simulink model "sim_track"  (Simulink 6.2)
settings: Solver=ode45  StartTime=0.0  StopTime=Tmax  MaxStep=0.01*T  RelTol=1e-6
undefined symbols (not defined in the file or in its folder): dF, dFo, dG, dK, dQ, dQu, dR, nF, nFo, nG, nK, nQ, nQu, nR, T, tauF, tauG, tauQ, tauQu, tauR
settings Model: LastModifiedBy=Administrator
settings DataIOCC: SignalLoggingName=sigsOut
settings OptimizationCC: BlockReduction=off  BooleanDataType=off  InlineInvariantSignals=on
settings HardwareCC: TargetUnknown=on

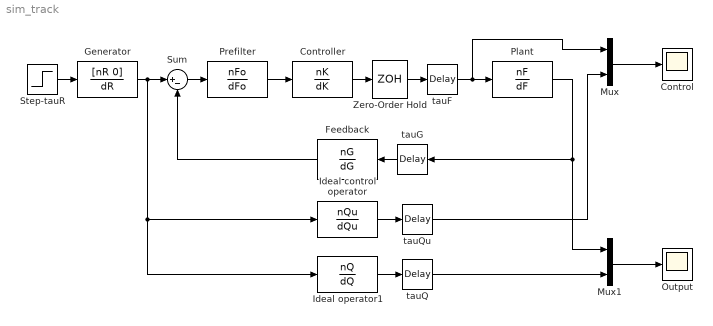
== system sim_track ==
  Control : Scope
      settings: TimeRange=10  YMin=0  YMax=2.1  SaveName=u  DataFormat=Array
  Controller : DiscreteTransferFcn  Numerator=nK  Denominator=dK  SampleTime=T
  Feedback : TransferFcn  Orientation=left  Numerator=nG  Denominator=dG
  Generator : TransferFcn  Numerator=[nR 0]  Denominator=dR
  Ideal control operator : TransferFcn  Numerator=nQu  Denominator=dQu
  Ideal operator1 : TransferFcn  Numerator=nQ  Denominator=dQ
  Mux : Mux  Inputs=2
  Mux1 : Mux  Inputs=2
  Output : Scope
      settings: TimeRange=50  YMin=0  YMax=14  SaveName=y  DataFormat=Array
  Plant : TransferFcn  Numerator=nF  Denominator=dF
  Prefilter : TransferFcn  Numerator=nFo  Denominator=dFo
  Step-tauR : Step  Time=tauR
  Sum : Sum  Inputs=|+-  SaturateOnIntegerOverflow=on  InputSameDT=on
  Zero-Order Hold : ZeroOrderHold  SampleTime=T
  tauF : TransportDelay  DelayTime=tauF  BufferSize=10240
  tauG : TransportDelay  Orientation=left  DelayTime=tauG  BufferSize=10240
  tauQ : TransportDelay  DelayTime=tauQ  BufferSize=10240
  tauQu : TransportDelay  DelayTime=tauQu  BufferSize=10240
  wires:
  Plant/1 -> Mux1/1, tauG/1
  Step-tauR/1 -> Generator/1
  Mux/1 -> Control/1
  Mux1/1 -> Output/1
  Ideal control operator/1 -> tauQu/1
  tauQu/1 -> Mux/2
  Ideal operator1/1 -> tauQ/1
  tauQ/1 -> Mux1/2
  Prefilter/1 -> Controller/1
  Controller/1 -> Zero-Order Hold/1
  Zero-Order Hold/1 -> tauF/1
  tauF/1 -> Mux/1, Plant/1
  Sum/1 -> Prefilter/1
  tauG/1 -> Feedback/1
  Feedback/1 -> Sum/2
  Generator/1 -> Sum/1, Ideal operator1/1, Ideal control operator/1
